simulink model "sampleModel142"  (R2021b)
settings: Solver=VariableStepAuto  StartTime=0.0  StopTime=10.0  RelTol=1e-3
undefined symbols (not defined in the file or in its folder): Newton, Raphson
libraries: simulink x4
settings Model: Creator=user  LastModifiedBy=user

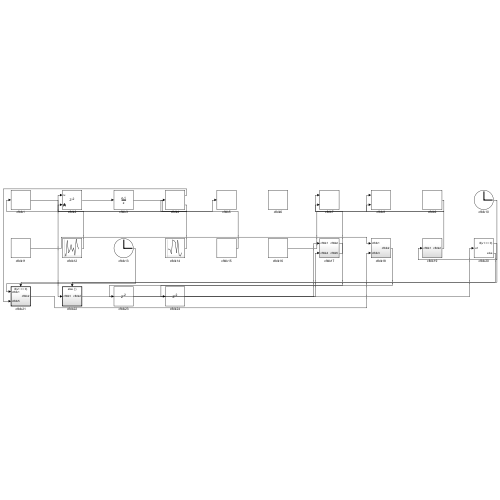
[thumbnail: Simulink's stored preview of the top-level diagram]
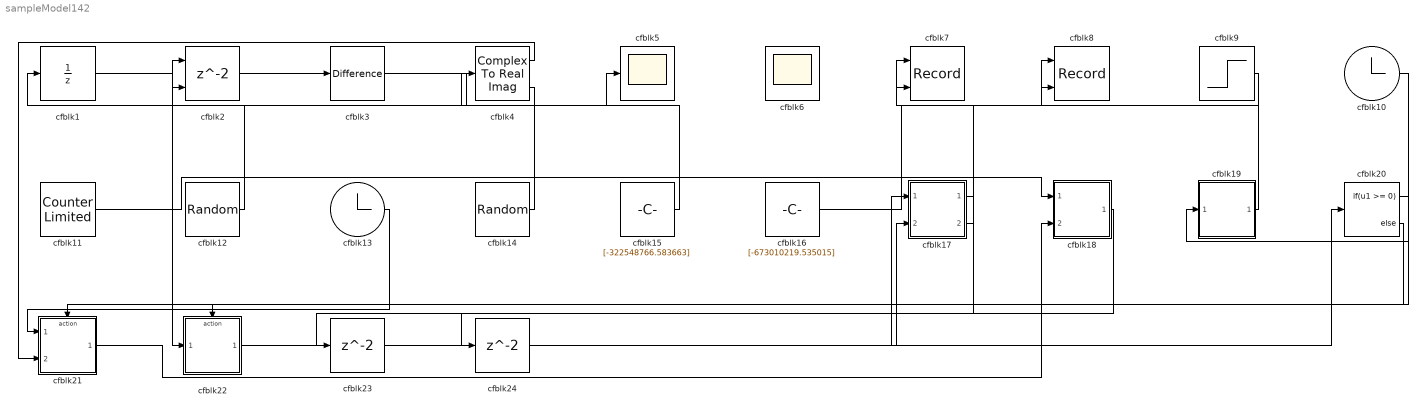
== system sampleModel142 ==
  cfblk1 : UnitDelay  HasFrameUpgradeWarning=on
  cfblk10 : Clock
  cfblk11 : simulink/Sources/Counter Limited  uplimit=[258.000000]  tsamp=-1
  cfblk12 : UniformRandomNumber  Minimum=[-8333604584.276587]  Maximum=[4403446205.768578]  Seed=[18033100.000000]  SampleTime=0.1
  cfblk13 : Clock
  cfblk14 : RandomNumber  Mean=[-85676.971278]  Variance=[37777.208341]  Seed=[449411398.000000]  SampleTime=0.1
  cfblk15 : Constant  Value=[-322548766.583663]  SampleTime=1
  cfblk16 : Constant  Value=[-673010219.535015]  SampleTime=1
  cfblk17 : Subsystem
  cfblk18 : Subsystem
  cfblk19 : Subsystem
  cfblk2 : Delay  ShowEnablePort=on  SampleTime=1
      settings: InputPortMap=u0,e6
  cfblk20 : If  IfExpression=u1 >= 0  SampleTime=1
  cfblk21 : Subsystem  TreatAsAtomicUnit=on
  cfblk22 : Subsystem  TreatAsAtomicUnit=on
  cfblk23 : Delay  SampleTime=1
  cfblk24 : Delay  SampleTime=1
  cfblk3 : simulink/Discrete/Difference  ICPrevInput=0.0  OutMin=[]  OutMax=[]  OutDataTypeStr=Inherit: Inherit via back propagation  OutDataType=fixdt(1, 16)  OutScaling=2^-10  DoSatur=off
  cfblk4 : ComplexToRealImag
  cfblk5 : Scope
  cfblk6 : Scope
      settings: Floating=on
  cfblk7 : Record  FileSettingsInternal="{\"entries\":[{\"content\":{\"excelSettings\":{\"content\":{},\"type\":\"Streamout.ExcelSettings\"}},\"type\":\"Streamout.FileSettingStorage\",\"uuid\":\"5c71d447-f7da-4f7c-b588-233883b38dc8\"}],\"packageUris\":[\"http://schema.mathworks.com/mf0/streamout_blocks/R2020a\"],\"version\":\"1.0\"}"  Layout=[1 1]  SignalsInternal="{\"entries\":[{\"content\":{\"signals\":[{\"content\":{\"blockPath\":[\"sampleModel142/cfblk7\"],\"channel\":[],\"dimensions\":[1],\"domain\":\"sampleModel142/cfblk7\",\"lineColor\":\"#a2142f\",\"plots\":[1],\"port\":1,\"sid\":[\"\"],\"signalID\":5084,\"signalName\":\"cfblk19\"},\"type\":\"RecordBlkView.Signal\",\"uuid\":\"97ec9cb9-f7b3-439a-8cdd-f76885870326\"},{\"content\":{\"blockPath\":[\"sampleModel142/cfblk7\"],\"channel\":[],\"dimensions\":[1],\"domain\":\"sampleModel142/cfblk7\",\"lineColor\":\"#139fff\",\"plots\":[1],\"port\":2,\"sid\":[\"\"],\"signalID\":5088,\"signalName\":\"cfblk17:2\"},\"type\":\"RecordBlkView.Signal\",\"uuid\":\"23ce8c57-8524-4c62-a008-c6e8e2d2d666\"}]},\"type\":\"RecordBlkView.InputSignals\",\"uuid\":\"45710655-93ab-44d0-bce8-dc9085c0d909\"}],\"packageUris\":[\"http://schema.mathworks.com/mf0/streamout_blocks/R2020a\"],\"version\":\"1.0\"}"  VisualizationBindings="{\"xyplotplugin\":{\"info\":[{\"series\":[{\"bindingParametersList\":[{\"parameter\":\"X-Axis\",\"signalID\":5084,\"signalName\":\"cfblk19\"},{\"parameter\":\"Y-Axis\",\"signalID\":5088,\"signalName\":\"cfblk17:2\"}],\"seriesID\":5101}],\"subplotID\":1}]}}"  CompatibilityTag=XY
  cfblk8 : Record  FileSettingsInternal="{\"entries\":[{\"content\":{\"excelSettings\":{\"content\":{},\"type\":\"Streamout.ExcelSettings\"}},\"type\":\"Streamout.FileSettingStorage\",\"uuid\":\"71c9d5a3-c152-467a-b858-d0dacf1fa973\"}],\"packageUris\":[\"http://schema.mathworks.com/mf0/streamout_blocks/R2020a\"],\"version\":\"1.0\"}"  Layout=[1 1]  SignalsInternal="{\"entries\":[{\"content\":{\"signals\":[{\"content\":{\"blockPath\":[\"sampleModel142/cfblk8\"],\"channel\":[],\"dimensions\":[1],\"domain\":\"sampleModel142/cfblk8\",\"lineColor\":\"#a2142f\",\"plots\":[1],\"port\":1,\"sid\":[\"\"],\"signalID\":5092,\"signalName\":\"cfblk16\"},\"type\":\"RecordBlkView.Signal\",\"uuid\":\"f4abf7b8-dd59-415d-a572-516493bc83e6\"},{\"content\":{\"blockPath\":[\"sampleModel142/cfblk8\"],\"channel\":[],\"dimensions\":[1],\"domain\":\"sampleModel142/cfblk8\",\"lineColor\":\"#139fff\",\"plots\":[1],\"port\":2,\"sid\":[\"\"],\"signalID\":5096,\"signalName\":\"cfblk9\"},\"type\":\"RecordBlkView.Signal\",\"uuid\":\"f031b583-1801-4665-82bc-3921c245e666\"}]},\"type\":\"RecordBlkView.InputSignals\",\"uuid\":\"072f772b-01b4-4bf0-bd07-b70d1ab3b8b6\"}],\"packageUris\":[\"http://schema.mathworks.com/mf0/streamout_blocks/R2020a\"],\"version\":\"1.0\"}"  VisualizationBindings="{\"xyplotplugin\":{\"info\":[{\"series\":[{\"bindingParametersList\":[{\"parameter\":\"X-Axis\",\"signalID\":5092,\"signalName\":\"cfblk16\"},{\"parameter\":\"Y-Axis\",\"signalID\":5096,\"signalName\":\"cfblk9\"}],\"seriesID\":27610}],\"subplotID\":1}]}}"  CompatibilityTag=XY
  cfblk9 : Step  Time=[2.000000]  Before=[896019277.368036]  After=[137868448.767294]  SampleTime=0
  wires:
  cfblk11/1 -> cfblk18/1(cfblk1)
  cfblk1/1 -> cfblk22/1(cfblk1)
  cfblk21/1(cfblk2) -> cfblk18/2(cfblk3)
  cfblk2/1 -> cfblk3/1
  cfblk13/1 -> cfblk21/1(cfblk1)
  cfblk12/1 -> cfblk1/1
  cfblk10/1 -> cfblk19/1(cfblk1)
  cfblk16/1 -> cfblk8/1
  cfblk22/1(cfblk2) -> cfblk17/2(cfblk4)
  cfblk19/1(cfblk2) -> cfblk7/1
  cfblk4/1 -> cfblk21/2(cfblk5)
  cfblk3/1 -> cfblk5/1
  cfblk15/1 -> cfblk2/1
  cfblk4/2 -> cfblk2/2
  cfblk14/1 -> cfblk4/1
  cfblk9/1 -> cfblk8/2
  cfblk17/2(cfblk5) -> cfblk7/2
  cfblk20/1 -> cfblk21/Action
  cfblk20/2 -> cfblk22/Action
  cfblk18/1(cfblk2) -> cfblk23/1
  cfblk23/1 -> cfblk17/1(cfblk1)
  cfblk17/1(cfblk2) -> cfblk24/1
  cfblk24/1 -> cfblk20/1

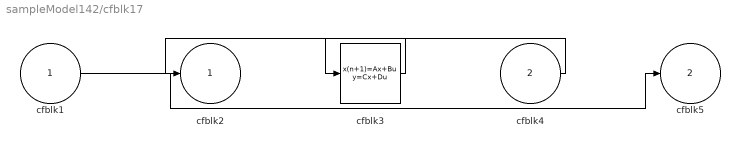
== system sampleModel142/cfblk17 ==
  cfblk1 : Inport
  cfblk4 : Inport  Port=2
  cfblk3 : DiscreteStateSpace
  cfblk2 : Outport
  cfblk5 : Outport  Port=2
  wires:
  cfblk4/1 -> cfblk3/1
  cfblk1/1 -> cfblk5/1
  cfblk3/1 -> cfblk2/1

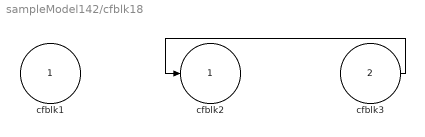
== system sampleModel142/cfblk18 ==
  cfblk1 : Inport
  cfblk3 : Inport  Port=2
  cfblk2 : Outport
  wires:
  cfblk3/1 -> cfblk2/1

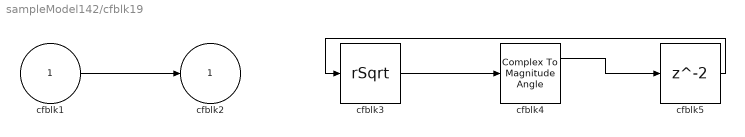
== system sampleModel142/cfblk19 ==
  cfblk1 : Inport
  cfblk3 : Sqrt  Operator=rSqrt  AlgorithmType=Newton-Raphson  SaturateOnIntegerOverflow=on
  cfblk4 : ComplexToMagnitudeAngle
  cfblk5 : Delay  SampleTime=1
  cfblk2 : Outport
  wires:
  cfblk1/1 -> cfblk2/1
  cfblk3/1 -> cfblk4/1
  cfblk4/1 -> cfblk5/1
  cfblk5/1 -> cfblk3/1

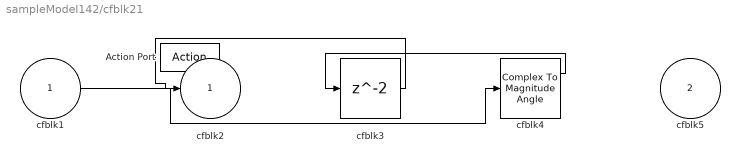
== system sampleModel142/cfblk21 ==
  cfblk1 : Inport
  cfblk5 : Inport  Port=2
  Action Port : ActionPort  ActionPortLabel=if(u1 >= 0)
  cfblk3 : Delay
  cfblk4 : ComplexToMagnitudeAngle
  cfblk2 : Outport
  wires:
  cfblk1/1 -> cfblk4/1
  cfblk3/1 -> cfblk2/1
  cfblk4/1 -> cfblk3/1

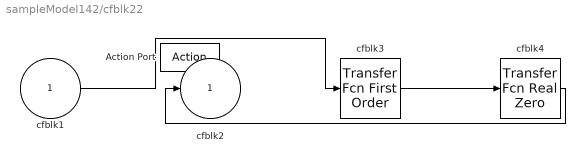
== system sampleModel142/cfblk22 ==
  cfblk1 : Inport
  Action Port : ActionPort  ActionPortLabel=else
  cfblk3 : simulink/Discrete/Transfer Fcn First Order  PoleZ=0.95  ICPrevOutput=0.0  DoSatur=off
  cfblk4 : simulink/Discrete/Transfer Fcn Real Zero  ZeroZ=0.75  ICPrevInput=0.0  DoSatur=off
      settings: SourceProductBaseCode=SL
  cfblk2 : Outport
  wires:
  cfblk4/1 -> cfblk2/1
  cfblk1/1 -> cfblk3/1
  cfblk3/1 -> cfblk4/1
